simulink model "ejercicio61"  (R2024a)
settings: Solver=VariableStepAuto  StartTime=0.0  StopTime=10.0  RelTol=1e-3
settings Model: Creator=Monsty  LastModifiedBy=Monsty

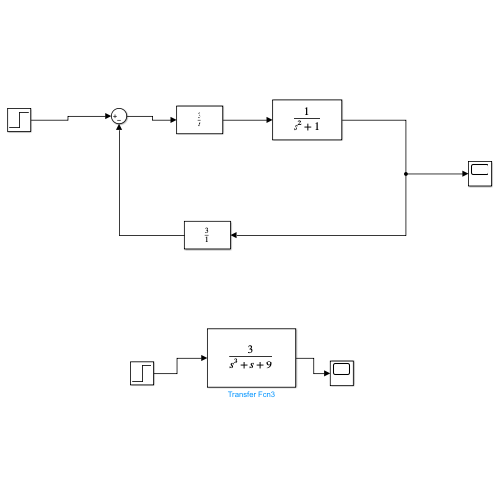
[thumbnail: Simulink's stored preview of the top-level diagram]
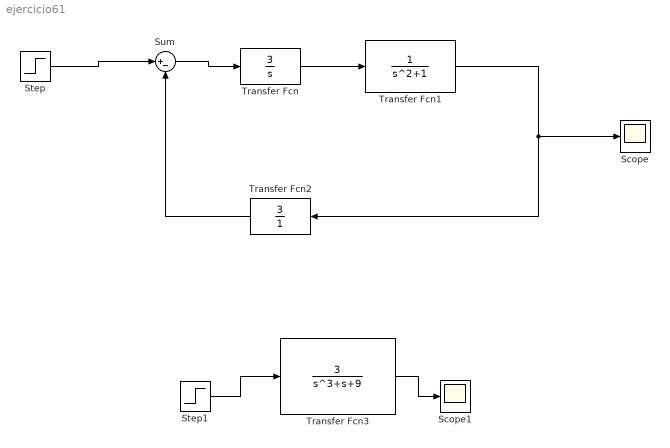
== system ejercicio61 ==
  Scope : Scope
  Scope1 : Scope
  Step : Step  SampleTime=0
  Step1 : Step  SampleTime=0
  Sum : Sum  Inputs=|+-
  Transfer Fcn : TransferFcn  Numerator=3  Denominator=[1 0]
  Transfer Fcn1 : TransferFcn  Denominator=[1 0 1]
  Transfer Fcn2 : TransferFcn  Numerator=[3]  Denominator=1
  Transfer Fcn3 : TransferFcn  Numerator=[3]  Denominator=[1 0 1 9]
  wires:
  Transfer Fcn/1 -> Transfer Fcn1/1
  Sum/1 -> Transfer Fcn/1
  Step/1 -> Sum/1
  Transfer Fcn1/1 -> Transfer Fcn2/1, Scope/1
  Transfer Fcn2/1 -> Sum/2
  Step1/1 -> Transfer Fcn3/1
  Transfer Fcn3/1 -> Scope1/1
